simulink model "cartesian_trajectory_planner_2"  (R2020a)
settings: Solver=FixedStepAuto  StartTime=0.0  StopTime=inf  FixedStep=0.05  RelTol=1e-3
libraries: robotlib x26, robotmaniplib x4, robotcorelib x3
settings Model: Creator=ROS_PO  LastModifiedBy=paolo
settings OptimizationCC: EnhancedBackFolding=on  PassReuseOutputArgsAs=Individual arguments  ZeroExternalMemoryAtStartup=off  ZeroInternalMemoryAtStartup=off  MaxStackSize=64  OptimizeBlockOrder=speed  DifferentSizesBufferReuse=on  OptimizationCustomize=off  EfficientTunableParamExpr=on
settings DebuggingCC: ParameterTunabilityLossMsg=error
settings HardwareCC: ProdBitPerPointer=32  ProdBitPerSizeT=32  ProdBitPerPtrDiffT=32  ProdLargestAtomicFloat=None  ProdIntDivRoundTo=Undefined  ProdEndianess=Unspecified  ProdWordSize=32  ProdHWDeviceType=Generic->Unspecified (assume 32-bit Generic)
settings RTWCC: SystemTargetFile=ert.tlc  HardwareBoard=Robot Operating System (ROS)  TemplateMakefile=ert_default_tmf  GenerateReport=on  Toolchain=Catkin  IncludeHyperlinkInReport=on  LaunchReport=on  TargetLang=C++  GenerateTraceInfo=on  GenerateTraceReport=on  GenerateTraceReportSl=on  GenerateTraceReportSf=on  GenerateTraceReportEml=on
settings CodeAppCC: ForceParamTrailComments=on  IgnoreCustomStorageClasses=off  OperatorAnnotations=on  SimulinkDataObjDesc=on  SFDataObjDesc=on  InsertBlockDesc=on
settings ERTTargetCC: SupportContinuousTime=on  SupportVariableSizeSignals=on

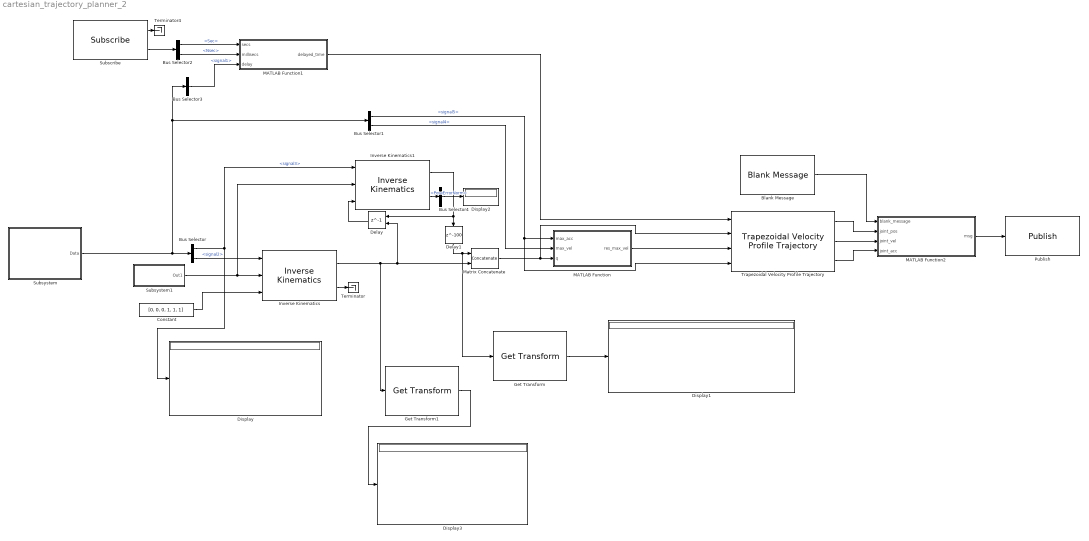
== system cartesian_trajectory_planner_2 ==
  Blank Message : robotlib/Blank Message  messageClass=Message  entityType=trajectory_msgs/JointTrajectoryPoint  messageType=trajectory_msgs/JointTrajectoryPoint  SampleTime=-1
  Bus Selector : BusSelector  OutputSignals=signal3,signal2
  Bus Selector1 : BusSelector  OutputSignals=signal5,signal4
  Bus Selector2 : BusSelector  OutputSignals=Clock_.Sec,Clock_.Nsec
  Bus Selector3 : BusSelector  OutputSignals=signal1
  Bus Selector4 : BusSelector  OutputSignals=PoseErrorNorm
  Constant : Constant  Value=[0, 0, 0, 1, 1, 1]
  Delay : Delay  DelayLength=1  InitialConditionSource=Input port  InitialCondition=[0, 0, 0, 0, 0, 0]
      settings: InputPortMap=u0,p4
  Delay1 : Delay  DelayLength=100  InitialCondition=zeros(6, 1, 100)
  Display{,1..3} (4 alike) : Display
  Get Transform : robotmaniplib/Get Transform  RigidBodyTree=robot  SourceBody=edo_link_ee  TargetBody=edo_base_link  SimulateUsing=Interpreted execution
  Get Transform1 : robotmaniplib/Get Transform  RigidBodyTree=robot  SourceBody=edo_link_ee  TargetBody=edo_base_link  SimulateUsing=Interpreted execution
  Inverse Kinematics : robotmaniplib/Inverse Kinematics  RigidBodyTree=robot  EndEffector=edo_link_ee  ShowInfo=on  SolverName=BFGS Gradient Projection  EnforceJointLimits=on  MaxIterations=1500  MaxTime=10  GradientTolerance=1e-7  SolutionTolerance=1e-6  StepTolerance=1e-14  ErrorChangeTolerance=1e-12  UseErrorDamping=on  DampingBias=0.0025  SimulateUsing=Interpreted execution
  Inverse Kinematics1 : robotmaniplib/Inverse Kinematics  RigidBodyTree=robot  EndEffector=edo_link_ee  ShowInfo=on  SolverName=BFGS Gradient Projection  EnforceJointLimits=on  MaxIterations=1500  MaxTime=10  GradientTolerance=1e-7  SolutionTolerance=1e-6  StepTolerance=1e-14  ErrorChangeTolerance=1e-12  UseErrorDamping=on  DampingBias=0.0025  SimulateUsing=Interpreted execution
  MATLAB Function : MATLAB Function  TreatAsAtomicUnit=on
  MATLAB Function1 : MATLAB Function  TreatAsAtomicUnit=on
  MATLAB Function2 : MATLAB Function  TreatAsAtomicUnit=on
  Matrix Concatenate : Concatenate  Mode=Multidimensional array  ConcatenateDimension=2
  Publish : robotlib/Publish  topicSource=Select from ROS network  topic=/joint_trajectory  messageType=trajectory_msgs/JointTrajectoryPoint  messageQueueLength=1
      link override SinkBlock: ROSTopic=/joint_trajectory  ROSMessageType=trajectory_msgs/JointTrajectoryPoint  SLBusName=SL_Bus_joint_trajectory_planner_JointTrajectoryPoint_y0wep  ModelName=joint_trajectory_planner  BlockId=Pub_joint_trajectory_planner_5
  Subscribe : robotlib/Subscribe  topicSource=Specify your own  topic=/clock  messageType=rosgraph_msgs/Clock  sampleTime=-1  messageQueueLength=1
  Subsystem : Subsystem
  Subsystem1 : Subsystem
  Terminator : Terminator
  Terminator4 : Terminator
  Trapezoidal Velocity Profile Trajectory : robotcorelib/Trapezoidal Velocity Profile Trajectory  WaypointSource=External  Waypoints=[ 0, -0.5, -1; 0, 0.5, 1 ]  NumParams=2  Parameter1=Peak Velocity  Parameter2=Acceleration  ParameterSource=External  PeakVelocity=[ 2; 2 ]  Acceleration=[ 1; 2 ]  EndTime=[ 1; 1 ]  AccelTime=[ 1; 2 ]  SimulateUsing=Interpreted execution
      settings: SourceProductBaseCode=NV,RO,RR
  wires:
  Inverse Kinematics/1 -> Get Transform1/1, Delay/2, Matrix Concatenate/2
  Bus Selector3/1 -> MATLAB Function1/3(delay)  "<signal1>"
  Subscribe/2 -> Bus Selector2/1
  Bus Selector1/1 -> Trapezoidal Velocity Profile Trajectory/4, MATLAB Function/1(max_acc)  "<signal5>"
  Inverse Kinematics/2 -> Terminator/1
  Trapezoidal Velocity Profile Trajectory/3 -> MATLAB Function2/4(joint_acc)
  Blank Message/1 -> MATLAB Function2/1(blank_message)
  Bus Selector2/1 -> MATLAB Function1/1(secs)  "<Sec>"
  Subscribe/1 -> Terminator4/1
  Inverse Kinematics1/2 -> Bus Selector4/1
  Bus Selector/1 -> Display/1, Inverse Kinematics1/1  "<signal3>"
  Constant/1 -> Inverse Kinematics/3
  Inverse Kinematics1/1 -> Delay1/1, Delay/1
  MATLAB Function/1(res_max_vel) -> Trapezoidal Velocity Profile Trajectory/3
  Bus Selector2/2 -> MATLAB Function1/2(millisecs)  "<Nsec>"
  MATLAB Function2/1(msg) -> Publish/1
  Bus Selector/2 -> Inverse Kinematics/1  "<signal2>"
  Trapezoidal Velocity Profile Trajectory/1 -> MATLAB Function2/2(joint_pos)
  Bus Selector1/2 -> MATLAB Function/2(max_vel)  "<signal4>"
  Trapezoidal Velocity Profile Trajectory/2 -> MATLAB Function2/3(joint_vel)
  Subsystem1/1(Out1) -> Inverse Kinematics1/2, Inverse Kinematics/2
  Subsystem/1(Data) -> Bus Selector3/1, Bus Selector1/1, Bus Selector/1
  MATLAB Function1/1(delayed_time) -> Trapezoidal Velocity Profile Trajectory/1
  Matrix Concatenate/1 -> Trapezoidal Velocity Profile Trajectory/2, MATLAB Function/3(q)
  Delay/1 -> Inverse Kinematics1/3
  Delay1/1 -> Get Transform/1, Matrix Concatenate/1
  Bus Selector4/1 -> Display2/1  "<PoseErrorNorm>"
  Get Transform/1 -> Display1/1
  Get Transform1/1 -> Display3/1

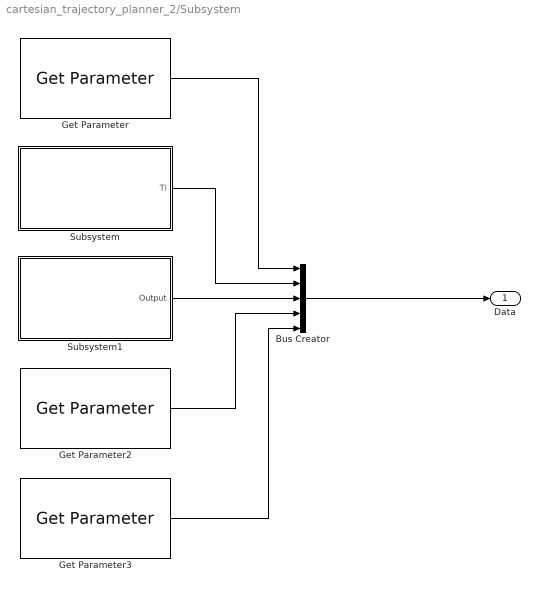
== system cartesian_trajectory_planner_2/Subsystem ==
  Bus Creator : BusCreator  Inputs=5
  Get Parameter : robotlib/Get Parameter  ParameterSource=Specify your own  ParameterName=/start_delay  ParameterType=double  ParameterMaxArrayLength=16  ParameterInitialValue=5.0  SampleTime=-1  ShowErrorCodeOutput=off  ModelName=cartesian_trajectory_planner_2  BlockId=ParamGet_cartesian_trajectory_planner_2_270
      settings: SourceProductBaseCode=RR
  Get Parameter2 : robotlib/Get Parameter  ParameterSource=Specify your own  ParameterName=/max_ang_vel  ParameterType=double  ParameterMaxArrayLength=16  ParameterInitialValue=1.0  SampleTime=-1  ShowErrorCodeOutput=off  ModelName=cartesian_trajectory_planner_2  BlockId=ParamGet_cartesian_trajectory_planner_2_271
      settings: SourceProductBaseCode=RR
  Get Parameter3 : robotlib/Get Parameter  ParameterSource=Specify your own  ParameterName=/max_ang_acc  ParameterType=double  ParameterMaxArrayLength=16  ParameterInitialValue=1.0  SampleTime=-1  ShowErrorCodeOutput=off  ModelName=cartesian_trajectory_planner_2  BlockId=ParamGet_cartesian_trajectory_planner_2_272
      settings: SourceProductBaseCode=RR
  Subsystem : Subsystem
  Subsystem1 : Subsystem
  Data : Outport
  wires:
  Subsystem/1(Ti) -> Bus Creator/2
  Bus Creator/1 -> Data/1
  Subsystem1/1(Output) -> Bus Creator/3
  Get Parameter2/1 -> Bus Creator/4
  Get Parameter3/1 -> Bus Creator/5
  Get Parameter/1 -> Bus Creator/1

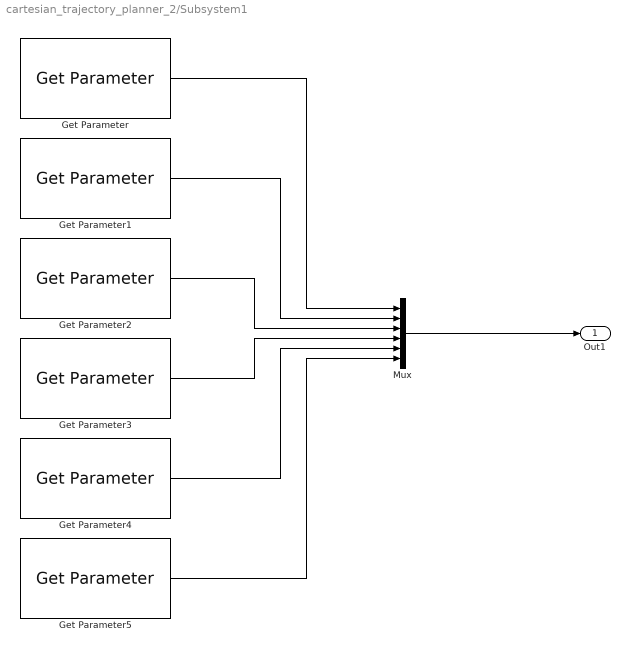
== system cartesian_trajectory_planner_2/Subsystem1 ==
  Get Parameter : robotlib/Get Parameter  ParameterSource=Specify your own  ParameterName=/weight_ox  ParameterType=double  ParameterMaxArrayLength=16  ParameterInitialValue=0  SampleTime=-1  ShowErrorCodeOutput=off  ModelName=cartesian_trajectory_planner_2  BlockId=ParamGet_cartesian_trajectory_planner_2_299
      settings: SourceProductBaseCode=RR
  Get Parameter1 : robotlib/Get Parameter  ParameterSource=Specify your own  ParameterName=/weight_oy  ParameterType=double  ParameterMaxArrayLength=16  ParameterInitialValue=0  SampleTime=-1  ShowErrorCodeOutput=off  ModelName=cartesian_trajectory_planner_2  BlockId=ParamGet_cartesian_trajectory_planner_2_300
      settings: SourceProductBaseCode=RR
  Get Parameter2 : robotlib/Get Parameter  ParameterSource=Specify your own  ParameterName=/weight_oz  ParameterType=double  ParameterMaxArrayLength=16  ParameterInitialValue=0  SampleTime=-1  ShowErrorCodeOutput=off  ModelName=cartesian_trajectory_planner_2  BlockId=ParamGet_cartesian_trajectory_planner_2_301
      settings: SourceProductBaseCode=RR
  Get Parameter3 : robotlib/Get Parameter  ParameterSource=Specify your own  ParameterName=/weight_px  ParameterType=double  ParameterMaxArrayLength=16  ParameterInitialValue=1  SampleTime=-1  ShowErrorCodeOutput=off  ModelName=cartesian_trajectory_planner_2  BlockId=ParamGet_cartesian_trajectory_planner_2_302
      settings: SourceProductBaseCode=RR
  Get Parameter4 : robotlib/Get Parameter  ParameterSource=Specify your own  ParameterName=/weight_py  ParameterType=double  ParameterMaxArrayLength=16  ParameterInitialValue=1  SampleTime=-1  ShowErrorCodeOutput=off  ModelName=cartesian_trajectory_planner_2  BlockId=ParamGet_cartesian_trajectory_planner_2_303
      settings: SourceProductBaseCode=RR
  Get Parameter5 : robotlib/Get Parameter  ParameterSource=Specify your own  ParameterName=/weight_pz  ParameterType=double  ParameterMaxArrayLength=16  ParameterInitialValue=1  SampleTime=-1  ShowErrorCodeOutput=off  ModelName=cartesian_trajectory_planner_2  BlockId=ParamGet_cartesian_trajectory_planner_2_304
      settings: SourceProductBaseCode=RR
  Mux : Mux  Inputs=6
  Out1 : Outport
  wires:
  Mux/1 -> Out1/1
  Get Parameter/1 -> Mux/1
  Get Parameter1/1 -> Mux/2
  Get Parameter2/1 -> Mux/3
  Get Parameter3/1 -> Mux/4
  Get Parameter4/1 -> Mux/5
  Get Parameter5/1 -> Mux/6

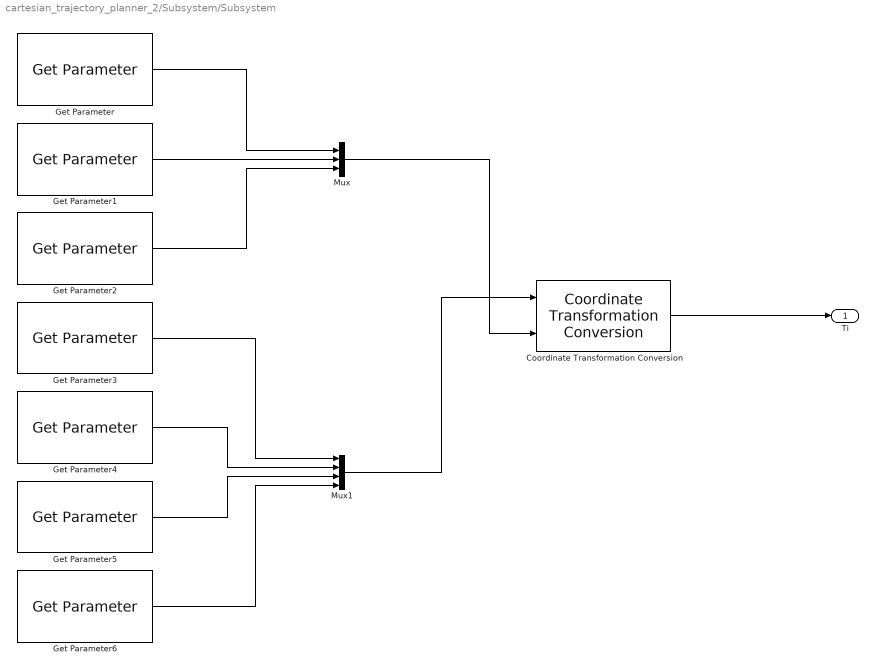
== system cartesian_trajectory_planner_2/Subsystem/Subsystem ==
  Coordinate Transformation Conversion : robotcorelib/Coordinate Transformation Conversion  InputRepresentation=Quaternion  InputEulerSequence=ZYX  ShowTrVecInputPort=on  OutputRepresentation=Homogeneous Transformation  OutputEulerSequence=ZYX  ShowTrVecOutputPort=on  SimulateUsing=Interpreted execution
      settings: SourceProductBaseCode=NV,RO,RR
  Get Parameter : robotlib/Get Parameter  ParameterSource=Specify your own  ParameterName=/pi_x  ParameterType=double  ParameterMaxArrayLength=16  ParameterInitialValue=0.0  SampleTime=-1  ShowErrorCodeOutput=off  ModelName=cartesian_trajectory_planner_2  BlockId=ParamGet_cartesian_trajectory_planner_2_275
      settings: SourceProductBaseCode=RR
  Get Parameter1 : robotlib/Get Parameter  ParameterSource=Specify your own  ParameterName=/pi_y  ParameterType=double  ParameterMaxArrayLength=16  ParameterInitialValue=0.0  SampleTime=-1  ShowErrorCodeOutput=off  ModelName=cartesian_trajectory_planner_2  BlockId=ParamGet_cartesian_trajectory_planner_2_276
      settings: SourceProductBaseCode=RR
  Get Parameter2 : robotlib/Get Parameter  ParameterSource=Specify your own  ParameterName=/pi_z  ParameterType=double  ParameterMaxArrayLength=16  ParameterInitialValue=0.99  SampleTime=-1  ShowErrorCodeOutput=off  ModelName=cartesian_trajectory_planner_2  BlockId=ParamGet_cartesian_trajectory_planner_2_277
      settings: SourceProductBaseCode=RR
  Get Parameter3 : robotlib/Get Parameter  ParameterSource=Specify your own  ParameterName=/oi_x  ParameterType=double  ParameterMaxArrayLength=16  ParameterInitialValue=0  SampleTime=-1  ShowErrorCodeOutput=off  ModelName=cartesian_trajectory_planner_2  BlockId=ParamGet_cartesian_trajectory_planner_2_278
      settings: SourceProductBaseCode=RR
  Get Parameter4 : robotlib/Get Parameter  ParameterSource=Specify your own  ParameterName=/oi_y  ParameterType=double  ParameterMaxArrayLength=16  ParameterInitialValue=0.0  SampleTime=-1  ShowErrorCodeOutput=off  ModelName=cartesian_trajectory_planner_2  BlockId=ParamGet_cartesian_trajectory_planner_2_279
      settings: SourceProductBaseCode=RR
  Get Parameter5 : robotlib/Get Parameter  ParameterSource=Specify your own  ParameterName=/oi_z  ParameterType=double  ParameterMaxArrayLength=16  ParameterInitialValue=0.0  SampleTime=-1  ShowErrorCodeOutput=off  ModelName=cartesian_trajectory_planner_2  BlockId=ParamGet_cartesian_trajectory_planner_2_280
      settings: SourceProductBaseCode=RR
  Get Parameter6 : robotlib/Get Parameter  ParameterSource=Specify your own  ParameterName=/oi_w  ParameterType=double  ParameterMaxArrayLength=16  ParameterInitialValue=1  SampleTime=-1  ShowErrorCodeOutput=off  ModelName=cartesian_trajectory_planner_2  BlockId=ParamGet_cartesian_trajectory_planner_2_281
      settings: SourceProductBaseCode=RR
  Mux : Mux  Inputs=3
  Mux1 : Mux
  Ti : Outport
  wires:
  Get Parameter/1 -> Mux/1
  Get Parameter1/1 -> Mux/2
  Get Parameter2/1 -> Mux/3
  Get Parameter3/1 -> Mux1/1
  Get Parameter4/1 -> Mux1/2
  Get Parameter5/1 -> Mux1/3
  Get Parameter6/1 -> Mux1/4
  Mux1/1 -> Coordinate Transformation Conversion/1
  Mux/1 -> Coordinate Transformation Conversion/2
  Coordinate Transformation Conversion/1 -> Ti/1

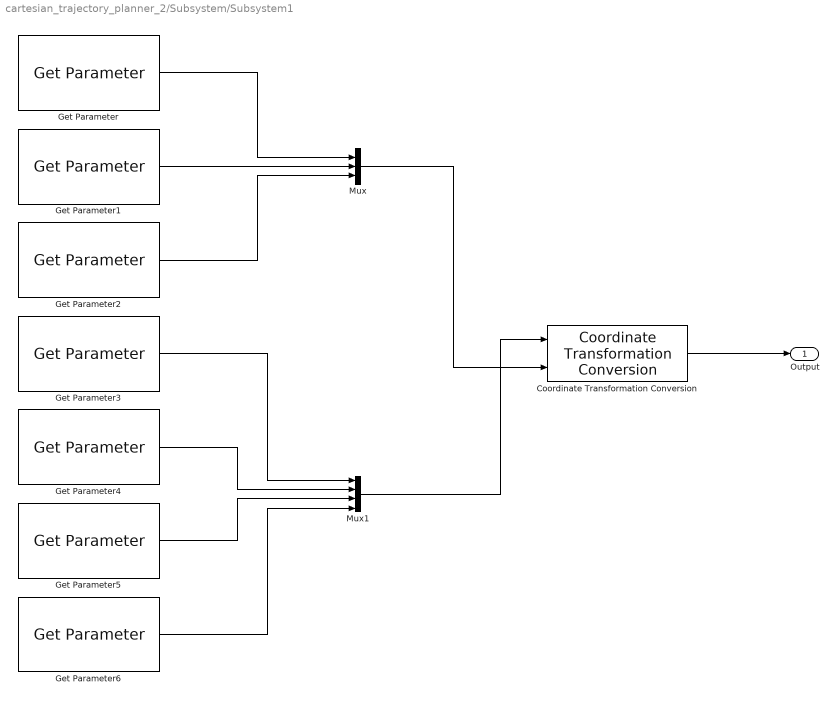
== system cartesian_trajectory_planner_2/Subsystem/Subsystem1 ==
  Coordinate Transformation Conversion : robotcorelib/Coordinate Transformation Conversion  InputRepresentation=Quaternion  InputEulerSequence=ZYX  ShowTrVecInputPort=on  OutputRepresentation=Homogeneous Transformation  OutputEulerSequence=ZYX  ShowTrVecOutputPort=on  SimulateUsing=Interpreted execution
      settings: SourceProductBaseCode=NV,RO,RR
  Get Parameter : robotlib/Get Parameter  ParameterSource=Specify your own  ParameterName=/pf_x  ParameterType=double  ParameterMaxArrayLength=16  ParameterInitialValue=0.3  SampleTime=-1  ShowErrorCodeOutput=off  ModelName=cartesian_trajectory_planner_2  BlockId=ParamGet_cartesian_trajectory_planner_2_287
      settings: SourceProductBaseCode=RR
  Get Parameter1 : robotlib/Get Parameter  ParameterSource=Specify your own  ParameterName=/pf_y  ParameterType=double  ParameterMaxArrayLength=16  ParameterInitialValue=0.3  SampleTime=-1  ShowErrorCodeOutput=off  ModelName=cartesian_trajectory_planner_2  BlockId=ParamGet_cartesian_trajectory_planner_2_288
      settings: SourceProductBaseCode=RR
  Get Parameter2 : robotlib/Get Parameter  ParameterSource=Specify your own  ParameterName=/pf_z  ParameterType=double  ParameterMaxArrayLength=16  ParameterInitialValue=0.3  SampleTime=-1  ShowErrorCodeOutput=off  ModelName=cartesian_trajectory_planner_2  BlockId=ParamGet_cartesian_trajectory_planner_2_289
      settings: SourceProductBaseCode=RR
  Get Parameter3 : robotlib/Get Parameter  ParameterSource=Specify your own  ParameterName=/of_x  ParameterType=double  ParameterMaxArrayLength=16  ParameterInitialValue=0.39  SampleTime=-1  ShowErrorCodeOutput=off  ModelName=cartesian_trajectory_planner_2  BlockId=ParamGet_cartesian_trajectory_planner_2_290
      settings: SourceProductBaseCode=RR
  Get Parameter4 : robotlib/Get Parameter  ParameterSource=Specify your own  ParameterName=/of_y  ParameterType=double  ParameterMaxArrayLength=16  ParameterInitialValue=0.89  SampleTime=-1  ShowErrorCodeOutput=off  ModelName=cartesian_trajectory_planner_2  BlockId=ParamGet_cartesian_trajectory_planner_2_291
      settings: SourceProductBaseCode=RR
  Get Parameter5 : robotlib/Get Parameter  ParameterSource=Specify your own  ParameterName=/of_z  ParameterType=double  ParameterMaxArrayLength=16  ParameterInitialValue=0.2  SampleTime=-1  ShowErrorCodeOutput=off  ModelName=cartesian_trajectory_planner_2  BlockId=ParamGet_cartesian_trajectory_planner_2_292
      settings: SourceProductBaseCode=RR
  Get Parameter6 : robotlib/Get Parameter  ParameterSource=Specify your own  ParameterName=/of_w  ParameterType=double  ParameterMaxArrayLength=16  ParameterInitialValue=-0.12  SampleTime=-1  ShowErrorCodeOutput=off  ModelName=cartesian_trajectory_planner_2  BlockId=ParamGet_cartesian_trajectory_planner_2_293
      settings: SourceProductBaseCode=RR
  Mux : Mux  Inputs=3
  Mux1 : Mux
  Output : Outport
  wires:
  Get Parameter/1 -> Mux/1
  Get Parameter1/1 -> Mux/2
  Get Parameter2/1 -> Mux/3
  Get Parameter3/1 -> Mux1/1
  Get Parameter4/1 -> Mux1/2
  Get Parameter5/1 -> Mux1/3
  Get Parameter6/1 -> Mux1/4
  Coordinate Transformation Conversion/1 -> Output/1
  Mux/1 -> Coordinate Transformation Conversion/2
  Mux1/1 -> Coordinate Transformation Conversion/1

== matlab function cartesian_trajectory_planner_2/MATLAB Function1 ==
  data: secs input; millisecs input; delay input; delayed_time output
function delayed_time = get_time(secs, millisecs, delay)

    time = secs + millisecs / 1e9;
    delayed_time = time - delay;
    
    if delayed_time < 0
        delayed_time = 0;
    end

== matlab function cartesian_trajectory_planner_2/MATLAB Function2 ==
  data: blank_message input; joint_pos input; msg output Bus: SL_Bus_cartesian_trajectory_plan_JointTrajectoryPoint_na5m06; joint_vel input; joint_acc input
function msg = assign_trajectory(blank_message, joint_pos, joint_vel, joint_acc)

    msg = blank_message;
    numJoints = length(joint_vel);
    msg.Velocities_SL_Info.CurrentLength = uint32(numJoints);
    msg.Velocities(1:numJoints) = joint_vel;
    msg.Positions_SL_Info.CurrentLength = uint32(numJoints);
    msg.Positions(1:numJoints) = joint_pos;
    msg.Accelerations_SL_Info.CurrentLength = uint32(numJoints);
    msg.Accelerations(1:numJoints) = joint_acc;

== matlab function cartesian_trajectory_planner_2/MATLAB Function ==
  data: max_acc input; max_vel input; q input; res_max_vel output
function res_max_vel = fcn(max_acc, max_vel, q)

    q_len = length(q);
    res_max_vel = max_vel * ones(q_len, 1);

    t_up = max_vel / max_acc;

    for i=1:q_len
        
        if abs(q(i,1)-q(i,2)) < max_vel * t_up
            res_max_vel(i) = abs(q(i,1) - q(i,2)) / t_up;
            
            if res_max_vel(i) == 0
                res_max_vel(i) = 0.01;
            end
        end

    end
